simulink model "model_2"  (R2018a)
settings: Solver=VariableStepAuto  StartTime=0.0  StopTime=10.0  RelTol=1e-3
values from neighbouring files (symbols this model uses):
  Af = 1.8    [script.m]
  Cd = 0.25    [script.m]
  fr = 0.015    [script.m]
  g = 9.81    [script.m]
  m_eq = delta*Mv    (= 1437.07)    [script.m]
  Mv = 1310    [script.m]
  rho = 1.2    [script.m]
libraries: simulink x1
settings Model: Creator=Saurabh Suman  LastModifiedBy=Saurabh Suman

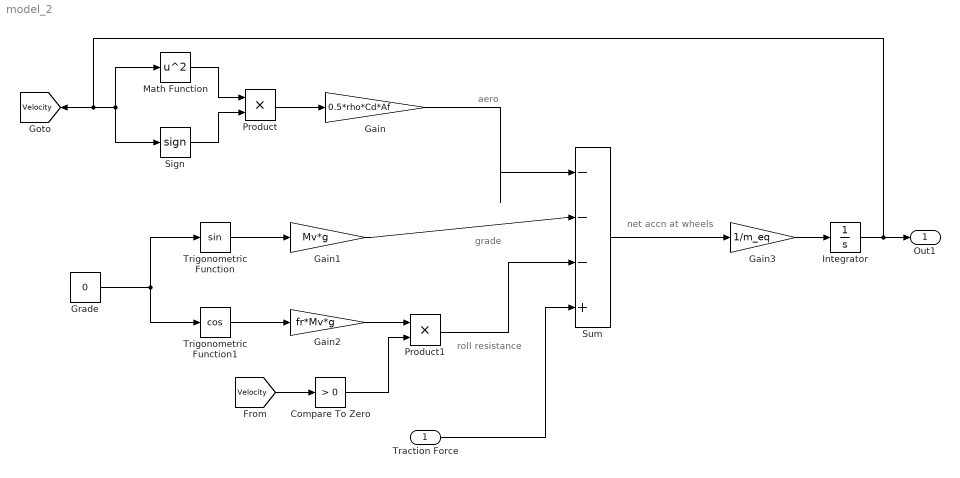
== system model_2 ==
  note: net accn at wheels
  note: roll resistance
  note: grade
  note: aero
  Traction Force : Inport
  Compare To Zero : simulink/Logic and Bit Operations/Compare To Zero  relop=>  OutDataTypeStr=boolean
  Gain : Gain  Gain=0.5*rho*Cd*Af
  Gain1 : Gain  Gain=Mv*g
  Gain2 : Gain  Gain=fr*Mv*g
  Gain3 : Gain  Gain=1/m_eq
  Grade : Constant  Value=0
  Integrator : Integrator
  Math Function : Math  Operator=square  SaturateOnIntegerOverflow=on
  Product : Product
  Product1 : Product
  Sign : Signum
  Sum : Sum  Inputs=|---+
  Trigonometric Function : Trigonometry
  Trigonometric Function1 : Trigonometry  Operator=cos
  Out1 : Outport
  tag scope: Velocity=global
  wires:
  Integrator/1 -> [Velocity], Sign/1, Math Function/1, Out1/1
  Math Function/1 -> Product/1
  Sign/1 -> Product/2
  Product/1 -> Gain/1
  Trigonometric Function1/1 -> Gain2/1
  Trigonometric Function/1 -> Gain1/1
  Grade/1 -> Trigonometric Function1/1, Trigonometric Function/1
  Gain2/1 -> Product1/1
  Compare To Zero/1 -> Product1/2
  [Velocity] -> Compare To Zero/1
  Gain/1 -> Sum/1
  Gain1/1 -> Sum/2
  Product1/1 -> Sum/3
  Sum/1 -> Gain3/1
  Traction Force/1 -> Sum/4
  Gain3/1 -> Integrator/1
